simulink model "TORALinearized"  (R2021a)
settings: Solver=VariableStepAuto  StartTime=0.0  StopTime=10.0  RelTol=1e-3
values from neighbouring files (symbols this model uses):
  A = [ 0 1      0 0 ... (first row only)    [epsysdyn.m]    (also in main_n10454012.m)
  B = [     0 ... (first row only)    [epsysdyn.m]    (also in main_n10454012.m)
  C = [ 0 0 0 0 ... (first row only)    [epsysdyn.m]    (also in kalmanfilter.m = [1 0 0 0]; main.m = [ 1 0 0 0; main_n10454012.m)
  controller_enabled = 1    [main.m]    (also in main_ClqrOkalmanI20deg0_1m.m; main_ClqrOoffI20deg0_1m.m; main_n10454012.m; maindefault.m)
  K = place(A, B, [l1, l2, l3, l4])    [kSearch.m]    (also in main.m = Klqr; main_ClqrOkalmanI20deg0_1m.m = Klqr; main_ClqrOoffI20deg0_1m.m = Klqr; main_n10454012.m = Klqr)
  L = 1    [initialise.m]    (also in main.m = Lnormal; main_ClqrOkalmanI20deg0_1m.m = Lkalman; main_ClqrOoffI20deg0_1m.m = Lkalman; main_n10454012.m = Lnormal)
  use_state_estimates = 1    [main.m]    (also in main_ClqrOkalmanI20deg0_1m.m; main_ClqrOoffI20deg0_1m.m = 0; main_n10454012.m; maindefault.m)
  x0 = [ 100*pi/180; 0; 0; 0 ]    [epsysdyn.m]    (also in main_n10454012.m = [ wrapTo180(20)*pi/180; 0; 0.1; 0 ])
  x_bar = xb_bar    [epsysdyn.m]    (also in main_n10454012.m)
settings Model: Creator=chilla  LastModifiedBy=chilla
settings SolverCC: AlgebraicLoopSolver=TrustRegion
settings DebuggingCC: SFMachineParentedDataDiag=warning

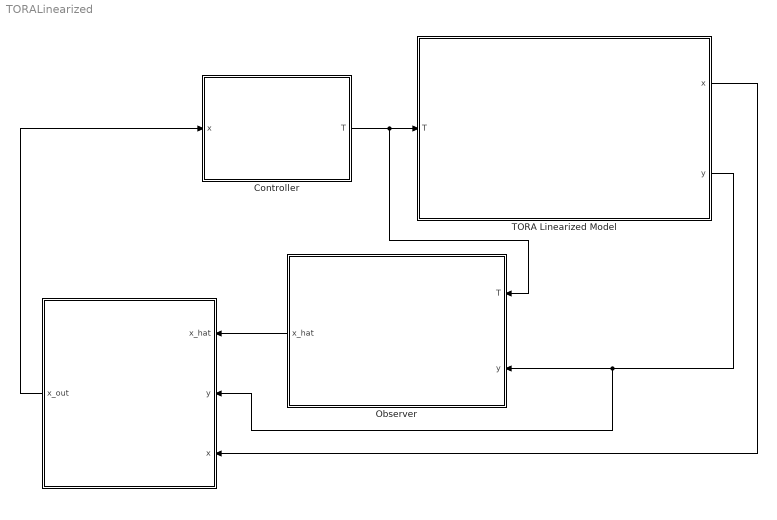
== system TORALinearized ==
  " " : Subsystem
  Controller : Subsystem
  Observer : Subsystem
  TORA Linearized Model : Subsystem
  wires:
  Controller/1(T) -> TORA Linearized Model/1(T), Observer/1(T)
  TORA Linearized Model/2(y) -> " "/2(y), Observer/2(y)
  TORA Linearized Model/1("x ") -> " "/3(x)
  Observer/1(x_hat) -> " "/1(x_hat)
  " "/1(x_out) -> Controller/1(x)

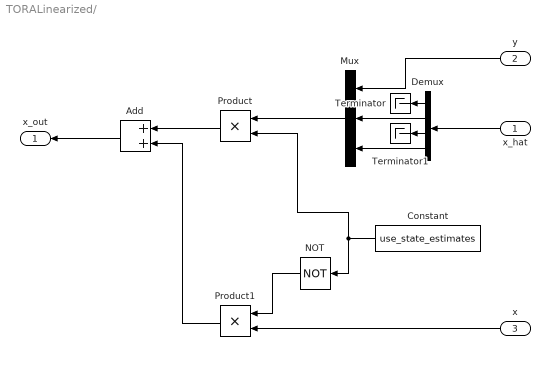
== system TORALinearized/  ==
  x_hat : Inport
  y : Inport  Port=2
  x : Inport  Port=3
  Add : Sum
  Constant : Constant  Value=use_state_estimates
  Demux : Demux
  Mux : Mux  Inputs=3
  NOT : Logic  Operator=NOT  IconShape=distinctive  AllPortsSameDT=off  OutDataTypeStr=boolean
  Product : Product
  Product1 : Product
  Terminator : Terminator
  Terminator1 : Terminator
  x_out : Outport
  wires:
  y/1 -> Mux/1
  x_hat/1 -> Demux/1
  Mux/1 -> Product/1
  Constant/1 -> Product/2, NOT/1
  x/1 -> Product1/2
  NOT/1 -> Product1/1
  Add/1 -> x_out/1
  Product/1 -> Add/1
  Product1/1 -> Add/2
  Demux/2 -> Mux/2
  Demux/4 -> Mux/3
  Demux/1 -> Terminator/1
  Demux/3 -> Terminator1/1

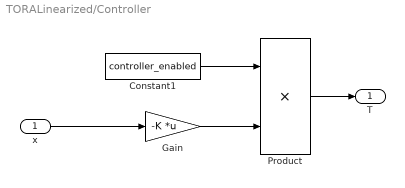
== system TORALinearized/Controller ==
  x : Inport
  Constant1 : Constant  Value=controller_enabled
  Gain : Gain  Gain=-K  Multiplication=Matrix(K*u)
  Product : Product
  T : Outport
  wires:
  x/1 -> Gain/1
  Product/1 -> T/1
  Constant1/1 -> Product/1
  Gain/1 -> Product/2

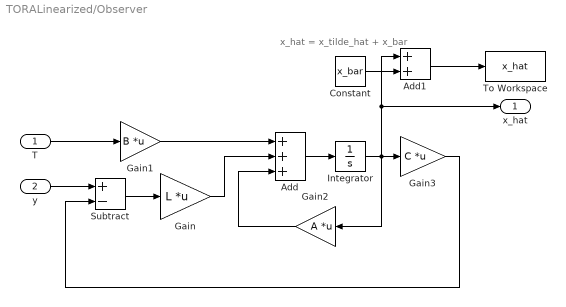
== system TORALinearized/Observer ==
  note: x_hat = x_tilde_hat + x_bar
  T : Inport
  y : Inport  Port=2
  Add : Sum  Inputs=+++
  Add1 : Sum
  Constant : Constant  Value=x_bar
  Gain : Gain  Gain=L  Multiplication=Matrix(K*u)
  Gain1 : Gain  Gain=B  Multiplication=Matrix(K*u)
  Gain2 : Gain  Gain=A  Multiplication=Matrix(K*u)
  Gain3 : Gain  Gain=C  Multiplication=Matrix(K*u)
  Integrator : Integrator
  Subtract : Sum  Inputs=+-
  To Workspace : ToWorkspace  VariableName=x_hat  SampleTime=-1
  x_hat : Outport  VectorParamsAs1DForOutWhenUnconnected=off
  wires:
  y/1 -> Subtract/1
  Subtract/1 -> Gain/1
  T/1 -> Gain1/1
  Gain1/1 -> Add/1
  Gain/1 -> Add/2
  Add/1 -> Integrator/1
  Gain2/1 -> Add/3
  Gain3/1 -> Subtract/2
  Integrator/1 -> x_hat/1, Add1/1, Gain2/1, Gain3/1
  Add1/1 -> To Workspace/1
  Constant/1 -> Add1/2

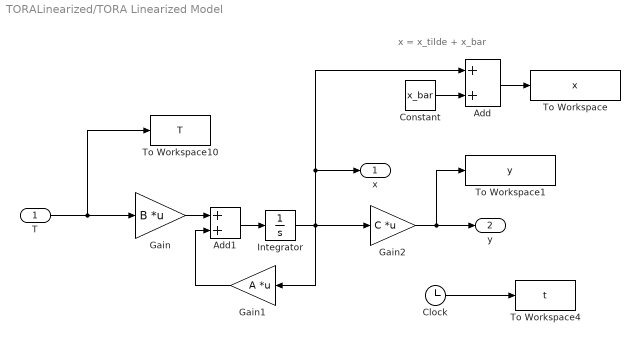
== system TORALinearized/TORA Linearized Model ==
  note: x = x_tilde + x_bar
  T : Inport
  Add : Sum
  Add1 : Sum
  Clock : Clock
  Constant : Constant  Value=x_bar
  Gain : Gain  Gain=B  Multiplication=Matrix(K*u)
  Gain1 : Gain  Gain=A  Multiplication=Matrix(K*u)
  Gain2 : Gain  Gain=C  Multiplication=Matrix(K*u)
  Integrator : Integrator  InitialCondition=x0-x_bar
  To Workspace : ToWorkspace  VariableName=x  SampleTime=-1
  To Workspace1 : ToWorkspace  VariableName=y  SampleTime=-1
  To Workspace10 : ToWorkspace  VariableName=T  SampleTime=-1
  To Workspace4 : ToWorkspace  VariableName=t  SampleTime=-1
  "x " : Outport  VectorParamsAs1DForOutWhenUnconnected=off
  y : Outport  Port=2  VectorParamsAs1DForOutWhenUnconnected=off
  wires:
  T/1 -> To Workspace10/1, Gain/1
  Gain/1 -> Add1/1
  Constant/1 -> Add/2
  Gain1/1 -> Add1/2
  Clock/1 -> To Workspace4/1
  Add1/1 -> Integrator/1
  Integrator/1 -> "x "/1, Add/1, Gain2/1, Gain1/1
  Add/1 -> To Workspace/1
  Gain2/1 -> To Workspace1/1, y/1
